simulink model "gm_case2mod_new"  (R2018b)
settings: Solver=FixedStepDiscrete  StartTime=0.0  StopTime=100000  FixedStep=1  RelTol=1e-3
(part 2 of 2)

== stateflow chart gm_case2mod_new/NA7_S2/node_aut/SimpleModeling_c4_sqCkIiGJ54r4u5oiueanYzC_node_aut ==
  settings: executeAtInitialization=1
  state NodeAutomaton
    state RRP
      du: TRRP_cur = TRRP_cur-1;
      du: state=3;
    state Rest
      du: Trest_cur = Trest_cur-1;
      du: state=1;
    state ERP
      ex: Active = 0;
      du: TERP_cur = TERP_cur-1;
      du: path_timer = 0;
      du: Active = 0;
      du: state=2;
    (default) -> Rest : {Active=0;
        | Trest_cur = Trest_s;TERP_def=TERP_defs;
        | TERP_cur = TERP_s;
        | TRRP_cur = TRRP_s;
        | path_timer = 0;}
    RRP -> Rest [order 2] : [(~inActive) & (TRRP_cur==0)]
        | {TRRP_cur = TRRP_def;
        | path_timer = 0;}
    Rest -> ERP [order 2] : [inActive]
        | {Trest_cur = Trest_def;
        | TERP_def = Terp_max;
        | TERP_cur = Terp_max;
        | path_timer = 1;}
    Rest -> ERP [order 1] : [(~inActive) & (Trest_cur==0)]
        | {Trest_cur = Trest_def;
        | Active = 1;
        | path_timer = 0;}
    RRP -> ERP [order 1] : [inActive]
        | {TERP_def = Terp_min;
        | path_timer = 3;
        | TERP_cur = TERP_def;
        | TRRP_cur = TRRP_def;}
    ERP -> RRP [order 2] : [(~inActive) & (TERP_cur==0)]
        | {TERP_cur = TERP_def;
        | path_timer = 0;}
    ERP -> ERP [order 1] : [inActive]
        | {TERP_cur = Terp_min;
        | TERP_def = Terp_min;
        | path_timer = 3;}
  data: TERP_cur local uint16; TRRP_cur local uint16; Trest_cur local uint16; TRRP_def constant uint16 =TRRP_def_m; Active output boolean; inActive input boolean; Trest_def input uint16 =Trest_def_m; TERP_defs constant uint16 =TERP_defs_m; TERP_s constant uint16 =TERP_s_m; TRRP_s constant uint16 =TRRP_s_m; Trest_s constant uint16 =Trest_s_m; Terp_min constant uint16 =Terp_min_m; Terp_max constant uint16 =Terp_max_m; TERP_def local uint16; state output uint8; path_timer output uint16; ratio local uint16

== stateflow chart gm_case2mod_new/PA1_1to2/path_aut/SimpleModeling_c5_sKnV4uZPaUgSl9dvj35Gf4B_path_aut ==
  settings: executeAtInitialization=1
  state PathAutomaton [parallel]
    settings: executionOrder=3
    state Idle
      en: idle_st = 1;
      du: state=1;
    state AntegradeConduction
      du: forw_timer_cur = forw_timer_cur-1;
      du: outActive1=0;
      du: idle_st = 0;
      du: state=2;
    state RetrogradeConduction
      du: bck_timer_cur = bck_timer_cur-1;
      du: outActive2=0;
      du: state=3;
    state Conflict
      ex: outActive2=0;
      ex: outActive1=0;
      du: state=4;
    state Double
      du: forw_timer_cur = forw_timer_cur-1;
      du: bck_timer_cur = bck_timer_cur-1;
      du: state=5;
    (default) -> Idle : {outActive1=0;
        | outActive2=0;}
    Idle -> AntegradeConduction [order 1] : [inActive1]
    Idle -> RetrogradeConduction [order 2] : [(~inActive1)&&(inActive2)]
    Conflict -> Idle
    RetrogradeConduction -> Conflict [order 1] : [bck_timer_cur==0 && (~inActive1)]
        | {bck_timer_cur=bck_timer_def;
        | outActive1=1;}
    AntegradeConduction -> Conflict [order 2] : [forw_timer_cur==0 && (~inActive2)]
        | {forw_timer_cur=forw_timer_def;
        | outActive2=1;}
    Double -> Conflict [order 2] : [(forw_timer_cur != 0) && (bck_timer_cur != 0)]
        | {forw_timer_cur=forw_timer_def;
        | bck_timer_cur=bck_timer_def;}
    Double -> RetrogradeConduction [order 3] : [forw_timer_cur==0]
        | {forw_timer_cur=forw_timer_def;
        | outActive2=1;}
    RetrogradeConduction -> Double [order 2] : [inActive1]
    AntegradeConduction -> Double [order 1] : [inActive2]
    Double -> AntegradeConduction [order 1] : [bck_timer_cur==0]
        | {bck_timer_cur=bck_timer_def;
        | outActive1=1;}
  state UpdateForward [parallel]
    settings: executionOrder=1
    state Update
    UpdateForward.Update -> UpdateForward.Update [order 1] : [(pathTimerEn > 0) && (idle_st)]
        | {forw_timer_def = forw_param * pathTimerEn;
        |  forw_timer_cur = forw_timer_def;}
    UpdateForward.Update -> UpdateForward.Update [order 2] : [(pathTimerEn > 0) && (~idle_st)]
        | {forw_timer_def = forw_param * pathTimerEn;}
  state UpdateBackward [parallel]
    settings: executionOrder=2
    state Update
    UpdateBackward.Update -> UpdateBackward.Update [order 1] : [(pathTimerEx > 0) && (idle_st)]
        | {bck_timer_def = bck_param * pathTimerEx;
        |  bck_timer_cur = bck_timer_def;}
    UpdateBackward.Update -> UpdateBackward.Update [order 2] : [(pathTimerEx > 0) && (~idle_st)]
        | {bck_timer_def = bck_param * pathTimerEx;}
  data: forw_timer_cur local uint16; bck_timer_cur local uint16; outActive1 output boolean; inActive1 input boolean; inActive2 input boolean; outActive2 output boolean; min_path_par constant uint16 =min_path_par_m; bck_timer_def local uint16; forw_timer_def local uint16; bck_param constant uint16 =bck_param_m; forw_param input uint16 =forw_param_m; idle_st local boolean; state output uint8; pathTimerEn input uint16; pathTimerEx input uint16

== stateflow chart gm_case2mod_new/PA2_2to3/path_aut/SimpleModeling_c5_spnshronzZ8815nA14cRtO_path_aut ==
  settings: executeAtInitialization=1
  state PathAutomaton [parallel]
    settings: executionOrder=3
    state Idle
      en: idle_st = 1;
      du: state=1;
    state AntegradeConduction
      du: forw_timer_cur = forw_timer_cur-1;
      du: outActive1=0;
      du: idle_st = 0;
      du: state=2;
    state RetrogradeConduction
      du: bck_timer_cur = bck_timer_cur-1;
      du: outActive2=0;
      du: state=3;
    state Conflict
      ex: outActive2=0;
      ex: outActive1=0;
      du: state=4;
    state Double
      du: forw_timer_cur = forw_timer_cur-1;
      du: bck_timer_cur = bck_timer_cur-1;
      du: state=5;
    (default) -> Idle : {outActive1=0;
        | outActive2=0;}
    Idle -> AntegradeConduction [order 1] : [inActive1]
    Idle -> RetrogradeConduction [order 2] : [(~inActive1)&&(inActive2)]
    Conflict -> Idle
    RetrogradeConduction -> Conflict [order 1] : [bck_timer_cur==0 && (~inActive1)]
        | {bck_timer_cur=bck_timer_def;
        | outActive1=1;}
    AntegradeConduction -> Conflict [order 2] : [forw_timer_cur==0 && (~inActive2)]
        | {forw_timer_cur=forw_timer_def;
        | outActive2=1;}
    Double -> Conflict [order 2] : [(forw_timer_cur != 0) && (bck_timer_cur != 0)]
        | {forw_timer_cur=forw_timer_def;
        | bck_timer_cur=bck_timer_def;}
    Double -> RetrogradeConduction [order 3] : [forw_timer_cur==0]
        | {forw_timer_cur=forw_timer_def;
        | outActive2=1;}
    RetrogradeConduction -> Double [order 2] : [inActive1]
    AntegradeConduction -> Double [order 1] : [inActive2]
    Double -> AntegradeConduction [order 1] : [bck_timer_cur==0]
        | {bck_timer_cur=bck_timer_def;
        | outActive1=1;}
  state UpdateForward [parallel]
    settings: executionOrder=1
    state Update
    UpdateForward.Update -> UpdateForward.Update [order 1] : [(pathTimerEn > 0) && (idle_st)]
        | {forw_timer_def = forw_param * pathTimerEn;
        |  forw_timer_cur = forw_timer_def;}
    UpdateForward.Update -> UpdateForward.Update [order 2] : [(pathTimerEn > 0) && (~idle_st)]
        | {forw_timer_def = forw_param * pathTimerEn;}
  state UpdateBackward [parallel]
    settings: executionOrder=2
    state Update
    UpdateBackward.Update -> UpdateBackward.Update [order 1] : [(pathTimerEx > 0) && (idle_st)]
        | {bck_timer_def = bck_param * pathTimerEx;
        |  bck_timer_cur = bck_timer_def;}
    UpdateBackward.Update -> UpdateBackward.Update [order 2] : [(pathTimerEx > 0) && (~idle_st)]
        | {bck_timer_def = bck_param * pathTimerEx;}
  data: forw_timer_cur local uint16; bck_timer_cur local uint16; outActive1 output boolean; inActive1 input boolean; inActive2 input boolean; outActive2 output boolean; min_path_par constant uint16 =min_path_par_m; bck_timer_def local uint16; forw_timer_def local uint16; bck_param constant uint16 =bck_param_m; forw_param input uint16 =forw_param_m; idle_st local boolean; state output uint8; pathTimerEn input uint16; pathTimerEx input uint16

== stateflow chart gm_case2mod_new/PA3_1to4/path_aut/SimpleModeling_c5_sLRpbKPPZaNK4eVsSRGul3D_path_aut ==
  settings: executeAtInitialization=1
  state PathAutomaton [parallel]
    settings: executionOrder=3
    state Idle
      en: idle_st = 1;
      du: state=1;
    state AntegradeConduction
      du: forw_timer_cur = forw_timer_cur-1;
      du: outActive1=0;
      du: idle_st = 0;
      du: state=2;
    state RetrogradeConduction
      du: bck_timer_cur = bck_timer_cur-1;
      du: outActive2=0;
      du: state=3;
    state Conflict
      ex: outActive2=0;
      ex: outActive1=0;
      du: state=4;
    state Double
      du: forw_timer_cur = forw_timer_cur-1;
      du: bck_timer_cur = bck_timer_cur-1;
      du: state=5;
    (default) -> Idle : {outActive1=0;
        | outActive2=0;}
    Idle -> AntegradeConduction [order 1] : [inActive1]
    Idle -> RetrogradeConduction [order 2] : [(~inActive1)&&(inActive2)]
    Conflict -> Idle
    RetrogradeConduction -> Conflict [order 1] : [bck_timer_cur==0 && (~inActive1)]
        | {bck_timer_cur=bck_timer_def;
        | outActive1=1;}
    AntegradeConduction -> Conflict [order 2] : [forw_timer_cur==0 && (~inActive2)]
        | {forw_timer_cur=forw_timer_def;
        | outActive2=1;}
    Double -> Conflict [order 2] : [(forw_timer_cur != 0) && (bck_timer_cur != 0)]
        | {forw_timer_cur=forw_timer_def;
        | bck_timer_cur=bck_timer_def;}
    Double -> RetrogradeConduction [order 3] : [forw_timer_cur==0]
        | {forw_timer_cur=forw_timer_def;
        | outActive2=1;}
    RetrogradeConduction -> Double [order 2] : [inActive1]
    AntegradeConduction -> Double [order 1] : [inActive2]
    Double -> AntegradeConduction [order 1] : [bck_timer_cur==0]
        | {bck_timer_cur=bck_timer_def;
        | outActive1=1;}
  state UpdateForward [parallel]
    settings: executionOrder=1
    state Update
    UpdateForward.Update -> UpdateForward.Update [order 1] : [(pathTimerEn > 0) && (idle_st)]
        | {forw_timer_def = forw_param * pathTimerEn;
        |  forw_timer_cur = forw_timer_def;}
    UpdateForward.Update -> UpdateForward.Update [order 2] : [(pathTimerEn > 0) && (~idle_st)]
        | {forw_timer_def = forw_param * pathTimerEn;}
  state UpdateBackward [parallel]
    settings: executionOrder=2
    state Update
    UpdateBackward.Update -> UpdateBackward.Update [order 1] : [(pathTimerEx > 0) && (idle_st)]
        | {bck_timer_def = bck_param * pathTimerEx;
        |  bck_timer_cur = bck_timer_def;}
    UpdateBackward.Update -> UpdateBackward.Update [order 2] : [(pathTimerEx > 0) && (~idle_st)]
        | {bck_timer_def = bck_param * pathTimerEx;}
  data: forw_timer_cur local uint16; bck_timer_cur local uint16; outActive1 output boolean; inActive1 input boolean; inActive2 input boolean; outActive2 output boolean; min_path_par constant uint16 =min_path_par_m; bck_timer_def local uint16; forw_timer_def local uint16; bck_param constant uint16 =bck_param_m; forw_param input uint16 =forw_param_m; idle_st local boolean; state output uint8; pathTimerEn input uint16; pathTimerEx input uint16

== stateflow chart gm_case2mod_new/PA4_1to6/path_aut/SimpleModeling_c5_sKsWQe5Kdh9JFwwvtW0IE3D_path_aut ==
  settings: executeAtInitialization=1
  state PathAutomaton [parallel]
    settings: executionOrder=3
    state Idle
      en: idle_st = 1;
      du: state=1;
    state AntegradeConduction
      du: forw_timer_cur = forw_timer_cur-1;
      du: outActive1=0;
      du: idle_st = 0;
      du: state=2;
    state RetrogradeConduction
      du: bck_timer_cur = bck_timer_cur-1;
      du: outActive2=0;
      du: state=3;
    state Conflict
      ex: outActive2=0;
      ex: outActive1=0;
      du: state=4;
    state Double
      du: forw_timer_cur = forw_timer_cur-1;
      du: bck_timer_cur = bck_timer_cur-1;
      du: state=5;
    (default) -> Idle : {outActive1=0;
        | outActive2=0;}
    Idle -> AntegradeConduction [order 1] : [inActive1]
    Idle -> RetrogradeConduction [order 2] : [(~inActive1)&&(inActive2)]
    Conflict -> Idle
    RetrogradeConduction -> Conflict [order 1] : [bck_timer_cur==0 && (~inActive1)]
        | {bck_timer_cur=bck_timer_def;
        | outActive1=1;}
    AntegradeConduction -> Conflict [order 2] : [forw_timer_cur==0 && (~inActive2)]
        | {forw_timer_cur=forw_timer_def;
        | outActive2=1;}
    Double -> Conflict [order 2] : [(forw_timer_cur != 0) && (bck_timer_cur != 0)]
        | {forw_timer_cur=forw_timer_def;
        | bck_timer_cur=bck_timer_def;}
    Double -> RetrogradeConduction [order 3] : [forw_timer_cur==0]
        | {forw_timer_cur=forw_timer_def;
        | outActive2=1;}
    RetrogradeConduction -> Double [order 2] : [inActive1]
    AntegradeConduction -> Double [order 1] : [inActive2]
    Double -> AntegradeConduction [order 1] : [bck_timer_cur==0]
        | {bck_timer_cur=bck_timer_def;
        | outActive1=1;}
  state UpdateForward [parallel]
    settings: executionOrder=1
    state Update
    UpdateForward.Update -> UpdateForward.Update [order 1] : [(pathTimerEn > 0) && (idle_st)]
        | {forw_timer_def = forw_param * pathTimerEn;
        |  forw_timer_cur = forw_timer_def;}
    UpdateForward.Update -> UpdateForward.Update [order 2] : [(pathTimerEn > 0) && (~idle_st)]
        | {forw_timer_def = forw_param * pathTimerEn;}
  state UpdateBackward [parallel]
    settings: executionOrder=2
    state Update
    UpdateBackward.Update -> UpdateBackward.Update [order 1] : [(pathTimerEx > 0) && (idle_st)]
        | {bck_timer_def = bck_param * pathTimerEx;
        |  bck_timer_cur = bck_timer_def;}
    UpdateBackward.Update -> UpdateBackward.Update [order 2] : [(pathTimerEx > 0) && (~idle_st)]
        | {bck_timer_def = bck_param * pathTimerEx;}
  data: forw_timer_cur local uint16; bck_timer_cur local uint16; outActive1 output boolean; inActive1 input boolean; inActive2 input boolean; outActive2 output boolean; min_path_par constant uint16 =min_path_par_m; bck_timer_def local uint16; forw_timer_def local uint16; bck_param constant uint16 =bck_param_m; forw_param input uint16 =forw_param_m; idle_st local boolean; state output uint8; pathTimerEn input uint16; pathTimerEx input uint16

== stateflow chart gm_case2mod_new/PA5_4to5/path_aut/SimpleModeling_c5_s5eks8Qa0EkC2gggO4am9GG_path_aut ==
  settings: executeAtInitialization=1
  state PathAutomaton [parallel]
    settings: executionOrder=3
    state Idle
      en: idle_st = 1;
      du: state=1;
    state AntegradeConduction
      du: forw_timer_cur = forw_timer_cur-1;
      du: outActive1=0;
      du: idle_st = 0;
      du: state=2;
    state RetrogradeConduction
      du: bck_timer_cur = bck_timer_cur-1;
      du: outActive2=0;
      du: state=3;
    state Conflict
      ex: outActive2=0;
      ex: outActive1=0;
      du: state=4;
    state Double
      du: forw_timer_cur = forw_timer_cur-1;
      du: bck_timer_cur = bck_timer_cur-1;
      du: state=5;
    (default) -> Idle : {outActive1=0;
        | outActive2=0;}
    Idle -> AntegradeConduction [order 1] : [inActive1]
    Idle -> RetrogradeConduction [order 2] : [(~inActive1)&&(inActive2)]
    Conflict -> Idle
    RetrogradeConduction -> Conflict [order 1] : [bck_timer_cur==0 && (~inActive1)]
        | {bck_timer_cur=bck_timer_def;
        | outActive1=1;}
    AntegradeConduction -> Conflict [order 2] : [forw_timer_cur==0 && (~inActive2)]
        | {forw_timer_cur=forw_timer_def;
        | outActive2=1;}
    Double -> Conflict [order 2] : [(forw_timer_cur != 0) && (bck_timer_cur != 0)]
        | {forw_timer_cur=forw_timer_def;
        | bck_timer_cur=bck_timer_def;}
    Double -> RetrogradeConduction [order 3] : [forw_timer_cur==0]
        | {forw_timer_cur=forw_timer_def;
        | outActive2=1;}
    RetrogradeConduction -> Double [order 2] : [inActive1]
    AntegradeConduction -> Double [order 1] : [inActive2]
    Double -> AntegradeConduction [order 1] : [bck_timer_cur==0]
        | {bck_timer_cur=bck_timer_def;
        | outActive1=1;}
  state UpdateForward [parallel]
    settings: executionOrder=1
    state Update
    UpdateForward.Update -> UpdateForward.Update [order 1] : [(pathTimerEn > 0) && (idle_st)]
        | {forw_timer_def = forw_param * pathTimerEn;
        |  forw_timer_cur = forw_timer_def;}
    UpdateForward.Update -> UpdateForward.Update [order 2] : [(pathTimerEn > 0) && (~idle_st)]
        | {forw_timer_def = forw_param * pathTimerEn;}
  state UpdateBackward [parallel]
    settings: executionOrder=2
    state Update
    UpdateBackward.Update -> UpdateBackward.Update [order 1] : [(pathTimerEx > 0) && (idle_st)]
        | {bck_timer_def = bck_param * pathTimerEx;
        |  bck_timer_cur = bck_timer_def;}
    UpdateBackward.Update -> UpdateBackward.Update [order 2] : [(pathTimerEx > 0) && (~idle_st)]
        | {bck_timer_def = bck_param * pathTimerEx;}
  data: forw_timer_cur local uint16; bck_timer_cur local uint16; outActive1 output boolean; inActive1 input boolean; inActive2 input boolean; outActive2 output boolean; min_path_par constant uint16 =min_path_par_m; bck_timer_def local uint16; forw_timer_def local uint16; bck_param constant uint16 =bck_param_m; forw_param input uint16 =forw_param_m; idle_st local boolean; state output uint8; pathTimerEn input uint16; pathTimerEx input uint16

== stateflow chart gm_case2mod_new/PA6_6to7/path_aut/SimpleModeling_c5_s5XQ586iC6QEN0xQSpsem4E_path_aut ==
  settings: executeAtInitialization=1
  state PathAutomaton [parallel]
    settings: executionOrder=3
    state Idle
      en: idle_st = 1;
      du: state=1;
    state AntegradeConduction
      du: forw_timer_cur = forw_timer_cur-1;
      du: outActive1=0;
      du: idle_st = 0;
      du: state=2;
    state RetrogradeConduction
      du: bck_timer_cur = bck_timer_cur-1;
      du: outActive2=0;
      du: state=3;
    state Conflict
      ex: outActive2=0;
      ex: outActive1=0;
      du: state=4;
    state Double
      du: forw_timer_cur = forw_timer_cur-1;
      du: bck_timer_cur = bck_timer_cur-1;
      du: state=5;
    (default) -> Idle : {outActive1=0;
        | outActive2=0;}
    Idle -> AntegradeConduction [order 1] : [inActive1]
    Idle -> RetrogradeConduction [order 2] : [(~inActive1)&&(inActive2)]
    Conflict -> Idle
    RetrogradeConduction -> Conflict [order 1] : [bck_timer_cur==0 && (~inActive1)]
        | {bck_timer_cur=bck_timer_def;
        | outActive1=1;}
    AntegradeConduction -> Conflict [order 2] : [forw_timer_cur==0 && (~inActive2)]
        | {forw_timer_cur=forw_timer_def;
        | outActive2=1;}
    Double -> Conflict [order 2] : [(forw_timer_cur != 0) && (bck_timer_cur != 0)]
        | {forw_timer_cur=forw_timer_def;
        | bck_timer_cur=bck_timer_def;}
    Double -> RetrogradeConduction [order 3] : [forw_timer_cur==0]
        | {forw_timer_cur=forw_timer_def;
        | outActive2=1;}
    RetrogradeConduction -> Double [order 2] : [inActive1]
    AntegradeConduction -> Double [order 1] : [inActive2]
    Double -> AntegradeConduction [order 1] : [bck_timer_cur==0]
        | {bck_timer_cur=bck_timer_def;
        | outActive1=1;}
  state UpdateForward [parallel]
    settings: executionOrder=1
    state Update
    UpdateForward.Update -> UpdateForward.Update [order 1] : [(pathTimerEn > 0) && (idle_st)]
        | {forw_timer_def = forw_param * pathTimerEn;
        |  forw_timer_cur = forw_timer_def;}
    UpdateForward.Update -> UpdateForward.Update [order 2] : [(pathTimerEn > 0) && (~idle_st)]
        | {forw_timer_def = forw_param * pathTimerEn;}
  state UpdateBackward [parallel]
    settings: executionOrder=2
    state Update
    UpdateBackward.Update -> UpdateBackward.Update [order 1] : [(pathTimerEx > 0) && (idle_st)]
        | {bck_timer_def = bck_param * pathTimerEx;
        |  bck_timer_cur = bck_timer_def;}
    UpdateBackward.Update -> UpdateBackward.Update [order 2] : [(pathTimerEx > 0) && (~idle_st)]
        | {bck_timer_def = bck_param * pathTimerEx;}
  data: forw_timer_cur local uint16; bck_timer_cur local uint16; outActive1 output boolean; inActive1 input boolean; inActive2 input boolean; outActive2 output boolean; min_path_par constant uint16 =min_path_par_m; bck_timer_def local uint16; forw_timer_def local uint16; bck_param constant uint16 =bck_param_m; forw_param input uint16 =forw_param_m; idle_st local boolean; state output uint8; pathTimerEn input uint16; pathTimerEx input uint16

== stateflow chart gm_case2mod_new/PA7_5to7/path_aut/SimpleModeling_c5_sqcjkKS4oBcaRaS68Vk5pPE_path_aut ==
  settings: executeAtInitialization=1
  state PathAutomaton [parallel]
    settings: executionOrder=3
    state Idle
      en: idle_st = 1;
      du: state=1;
    state AntegradeConduction
      du: forw_timer_cur = forw_timer_cur-1;
      du: outActive1=0;
      du: idle_st = 0;
      du: state=2;
    state RetrogradeConduction
      du: bck_timer_cur = bck_timer_cur-1;
      du: outActive2=0;
      du: state=3;
    state Conflict
      ex: outActive2=0;
      ex: outActive1=0;
      du: state=4;
    state Double
      du: forw_timer_cur = forw_timer_cur-1;
      du: bck_timer_cur = bck_timer_cur-1;
      du: state=5;
    (default) -> Idle : {outActive1=0;
        | outActive2=0;}
    Idle -> AntegradeConduction [order 1] : [inActive1]
    Idle -> RetrogradeConduction [order 2] : [(~inActive1)&&(inActive2)]
    Conflict -> Idle
    RetrogradeConduction -> Conflict [order 1] : [bck_timer_cur==0 && (~inActive1)]
        | {bck_timer_cur=bck_timer_def;
        | outActive1=1;}
    AntegradeConduction -> Conflict [order 2] : [forw_timer_cur==0 && (~inActive2)]
        | {forw_timer_cur=forw_timer_def;
        | outActive2=1;}
    Double -> Conflict [order 2] : [(forw_timer_cur != 0) && (bck_timer_cur != 0)]
        | {forw_timer_cur=forw_timer_def;
        | bck_timer_cur=bck_timer_def;}
    Double -> RetrogradeConduction [order 3] : [forw_timer_cur==0]
        | {forw_timer_cur=forw_timer_def;
        | outActive2=1;}
    RetrogradeConduction -> Double [order 2] : [inActive1]
    AntegradeConduction -> Double [order 1] : [inActive2]
    Double -> AntegradeConduction [order 1] : [bck_timer_cur==0]
        | {bck_timer_cur=bck_timer_def;
        | outActive1=1;}
  state UpdateForward [parallel]
    settings: executionOrder=1
    state Update
    UpdateForward.Update -> UpdateForward.Update [order 1] : [(pathTimerEn > 0) && (idle_st)]
        | {forw_timer_def = forw_param * pathTimerEn;
        |  forw_timer_cur = forw_timer_def;}
    UpdateForward.Update -> UpdateForward.Update [order 2] : [(pathTimerEn > 0) && (~idle_st)]
        | {forw_timer_def = forw_param * pathTimerEn;}
  state UpdateBackward [parallel]
    settings: executionOrder=2
    state Update
    UpdateBackward.Update -> UpdateBackward.Update [order 1] : [(pathTimerEx > 0) && (idle_st)]
        | {bck_timer_def = bck_param * pathTimerEx;
        |  bck_timer_cur = bck_timer_def;}
    UpdateBackward.Update -> UpdateBackward.Update [order 2] : [(pathTimerEx > 0) && (~idle_st)]
        | {bck_timer_def = bck_param * pathTimerEx;}
  data: forw_timer_cur local uint16; bck_timer_cur local uint16; outActive1 output boolean; inActive1 input boolean; inActive2 input boolean; outActive2 output boolean; min_path_par constant uint16 =min_path_par_m; bck_timer_def local uint16; forw_timer_def local uint16; bck_param constant uint16 =bck_param_m; forw_param input uint16 =forw_param_m; idle_st local boolean; state output uint8; pathTimerEn input uint16; pathTimerEx input uint16

== stateflow chart gm_case2mod_new/PAC/SimpleModeling_c8_PVC ==
  settings: executeAtInitialization=1
  state Count
    du:PVC=0;
    du: count=count-1;
  state Wait
    du: PVC=0;
  state start
    du: PVC=0;
  Count -> Wait : [count==0]
      | {PVC=1;}
  (default) -> Wait
  start -> Count : [act==1]
      | {count=count_def;}
  Wait -> start : [st_en==1]
      | {}
  data: st_en input boolean; count_def input uint16; act input boolean; PVC output boolean; count local uint16

== stateflow chart gm_case2mod_new/PVC/SimpleModeling_c8_PVC ==
  settings: executeAtInitialization=1
  state Count
    du:PVC=0;
    du: count=count-1;
  state Wait
    du: PVC=0;
  state start
    du: PVC=0;
  Count -> Wait : [count==0]
      | {PVC=1;}
  (default) -> Wait
  start -> Count : [act==1]
      | {count=count_def;}
  Wait -> start : [st_en==1]
      | {}
  data: st_en input boolean; count_def input uint16; act input boolean; PVC output boolean; count local uint16
